simulink model "S_Function_StateSpaceControllerRobust"  (R2020b)
settings: Solver=VariableStepAuto  StartTime=0.0  StopTime=10.0  RelTol=1e-3
settings Model: Creator=Musta  LastModifiedBy=Musta

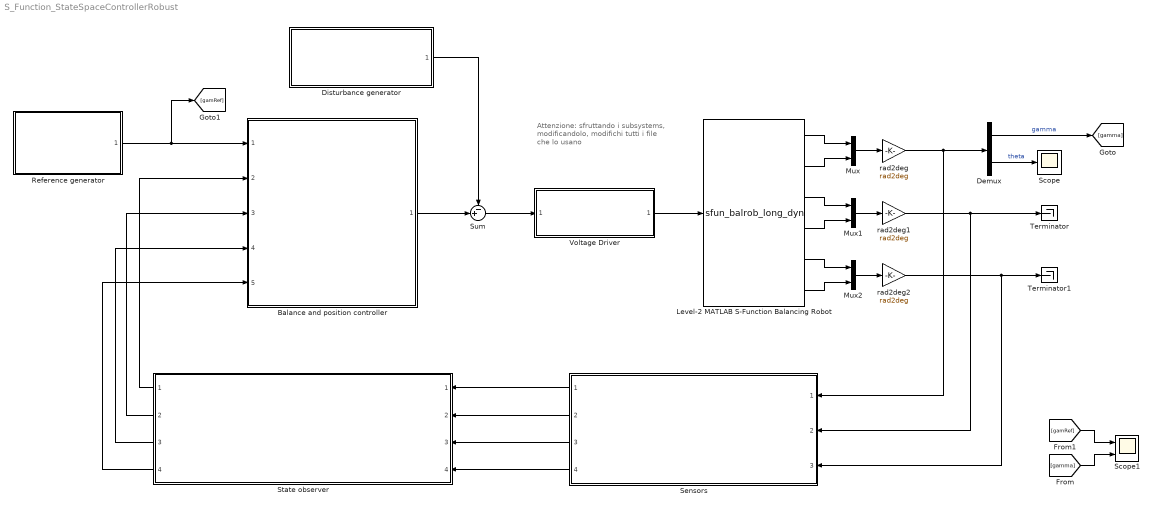
== system S_Function_StateSpaceControllerRobust ==
  note: Attenzione: sfruttando i subsystems, modificandolo, modifichi tutti i file che lo usano
  Balance and position controller : Subsystem  ReferencedSubsystem=StateSpaceControllerRobust_SubSystem
  Demux : Demux  Outputs=2
  Disturbance generator : Subsystem  ReferencedSubsystem=DisturbanceGenerator_SubSystem
  Level-2 MATLAB S-Function Balancing Robot : M-S-Function  FunctionName=sfun_balrob_long_dyn  Parameters=x0 body mot gbox wheel
  Mux : Mux  Inputs=2
  Mux1 : Mux  Inputs=2
  Mux2 : Mux  Inputs=2
  Reference generator : Subsystem  ReferencedSubsystem=GeneratorGam_ref_SubSystem
  Scope : Scope
  Scope1 : Scope  NumInputPorts=2
  Sensors : Subsystem  ReferencedSubsystem=Sensors_SubSystem
      settings: PortSchema="{\"entries\":[{\"content\":{\"sides\":[{\"content\":{\"connectorIds\":[\"Out1\",\"Out2\",\"Out3\",\"Out4\"]},\"type\":\"ConnectorPlacement.EquallySpacedRectSide\",\"uuid\":\"09d2c781-ae89-48e7-a59b-a0139f85cbb9\"},{\"content\":{\"connectorIds\":[\"In1\",\"In2\",\"In3\"],\"side\":\"RIGHT\"},\"type\":\"ConnectorPlacement.EquallySpacedRectSide\",\"uuid\":\"d911c94b-4df1-44da-afc4-33066bbfcbb9\"},{\"content\":{\"connectorIds\":[],\"side\":\"TOP\"},\"type\":\"ConnectorPlacement.EquallySpacedRectSide\",\"uuid\":\"3f014209-86c6-4281-b955-87c340eb85c4\"},{\"content\":{\"connectorIds\":[],\"side\":\"HIDDEN\"},\"type\":\"ConnectorPlacement.EquallySpacedRectSide\",\"uuid\":\"6e9e2372-5f7f-4905-b0ca-4299dfe2e7c3\"}]},\"type\":\"ConnectorPlacement.EquallySpacedConnector\",\"uuid\":\"4f7ca501-8ca2-46f3-9a27-b0b27745fee3\"}],\"packageUris\":[\"http://schema.mathworks.com/mf0/Connector/R2020b\"],\"version\":\"1.0\"}"
  State observer : Subsystem  ReferencedSubsystem=SimpleStateObserver_SubSystem
  Sum : Sum  Inputs=-+|
  Terminator : Terminator
  Terminator1 : Terminator
  Voltage Driver : Subsystem  ReferencedSubsystem=VoltageDriver_SubSystem
  rad2deg : Gain  Gain=rad2deg
  rad2deg1 : Gain  Gain=rad2deg
  rad2deg2 : Gain  Gain=rad2deg
  wires:
  Level-2 MATLAB S-Function Balancing Robot/2 -> Mux/2
  Level-2 MATLAB S-Function Balancing Robot/1 -> Mux/1
  Level-2 MATLAB S-Function Balancing Robot/3 -> Mux1/1
  Level-2 MATLAB S-Function Balancing Robot/4 -> Mux1/2
  Level-2 MATLAB S-Function Balancing Robot/6 -> Mux2/2
  Level-2 MATLAB S-Function Balancing Robot/5 -> Mux2/1
  Mux2/1 -> rad2deg2/1
  Mux1/1 -> rad2deg1/1
  Mux/1 -> rad2deg/1
  State observer/2 -> Balance and position controller/3
  Reference generator/1 -> [gamRef], Balance and position controller/1
  State observer/4 -> Balance and position controller/5
  Disturbance generator/1 -> Sum/1
  Sensors/1 -> State observer/1
  Sum/1 -> Voltage Driver/1
  State observer/3 -> Balance and position controller/4
  Sensors/4 -> State observer/4
  Sensors/3 -> State observer/3
  State observer/1 -> Balance and position controller/2
  Demux/1 -> [gamma]  "gamma"
  rad2deg/1 -> Demux/1, Sensors/1
  Voltage Driver/1 -> Level-2 MATLAB S-Function Balancing Robot/1
  Demux/2 -> Scope/1  "theta"
  Sensors/2 -> State observer/2
  rad2deg1/1 -> Terminator/1, Sensors/2
  rad2deg2/1 -> Terminator1/1, Sensors/3
  Balance and position controller/1 -> Sum/2
  [gamRef] -> Scope1/1
  [gamma] -> Scope1/2
